simulink model "fxpdemo_probe"  (Simulink 7.6)
settings: Solver=ode45  StartTime=0.0  StopTime=10.0  RelTol=1e-3
Description:
  | Fixed-Point S-Functions: Querying Properties
  | 
  | This model includes more than a dozen examples of S-functions used to probe signal properties.
  | Use this model for simulation only; it does not support code generation.
settings Model: Creator=The MathWorks Inc.  ExtModeAutoUpdateStatusClock=off
settings DataIOCC: SignalLoggingName=logsOut
settings OptimizationCC: InlineInvariantSignals=on  InitFltsAndDblsToZero=on
settings DebuggingCC: SignalResolutionControl=TryResolveAllWithWarning  SolverPrmCheckMsg=none  MultiTaskDSMMsg=warning  MultiTaskCondExecSysMsg=none  SigSpecEnsureSampleTimeMsg=none  StrictBusMsg=None
settings HardwareCC: TargetUnknown=on
settings RTWCC: IncludeERTFirstTime=on

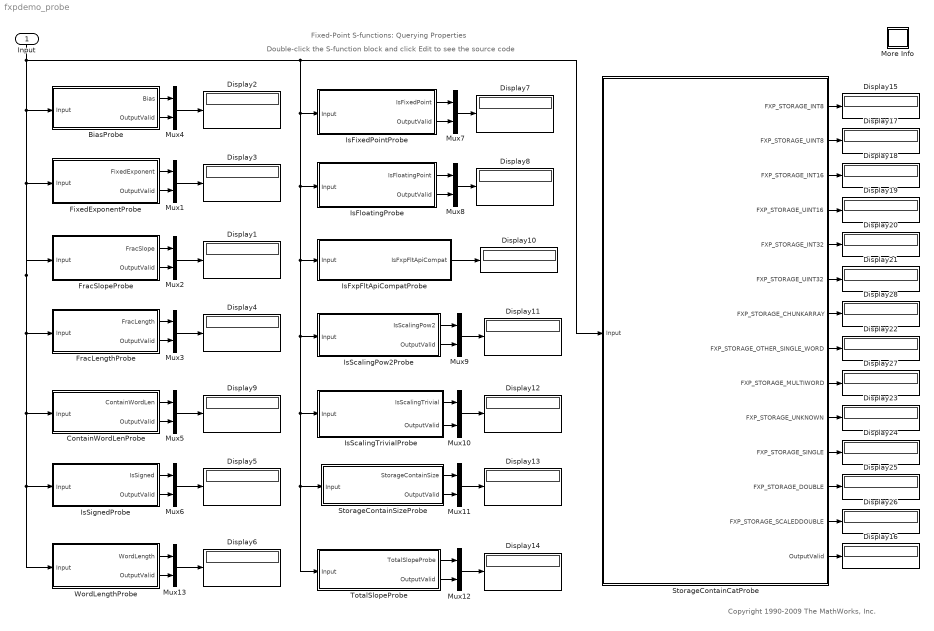
== system fxpdemo_probe ==
  note: Fixed-Point S-functions: Querying Properties
  note: Double-click the S-function block and click Edit to see the source code
  note: Copyright 1990-2009 The MathWorks, Inc.
  Input : Inport  OutDataTypeStr=fixdt(1, 33, 1.1*2^-3,10)
  BiasProbe : Subsystem
  ContainWordLenProbe : Subsystem
  Display{1..28} (28 alike) : Display
  FixedExponentProbe : Subsystem
  FracLengthProbe : Subsystem
  FracSlopeProbe : Subsystem
  IsFixedPointProbe : Subsystem
  IsFloatingProbe : Subsystem
  IsFxpFltApiCompatProbe : Subsystem
  IsScalingPow2Probe : Subsystem
  IsScalingTrivialProbe : Subsystem
  IsSignedProbe : Subsystem
  More Info : Subsystem
      settings: OpenFcn=showdemo(bdroot(gcs))
      mask Display: disp('?')
  Mux{1..13} (13 alike) : Mux  Inputs=2
  StorageContainCatProbe : Subsystem
  StorageContainSizeProbe : Subsystem
  "TotalSlopeProbe " : Subsystem
  WordLengthProbe : Subsystem
  wires:
  Mux5/1 -> Display9/1
  Mux3/1 -> Display4/1
  Mux2/1 -> Display1/1
  Mux1/1 -> Display3/1
  Mux4/1 -> Display2/1
  Input/1 -> FixedExponentProbe/1(Input), BiasProbe/1(Input), IsFixedPointProbe/1(Input), IsFloatingProbe/1(Input), IsFxpFltApiCompatProbe/1(Input), IsScalingPow2Probe/1(Input), IsScalingTrivialProbe/1(Input), StorageContainSizeProbe/1(Input), "TotalSlopeProbe "/1(Input), StorageContainCatProbe/1(Input), FracSlopeProbe/1(Input), FracLengthProbe/1(Input), ContainWordLenProbe/1(Input), IsSignedProbe/1(Input), WordLengthProbe/1(Input)
  Mux6/1 -> Display5/1
  IsSignedProbe/1(IsSigned) -> Mux6/1
  IsSignedProbe/2(OutputValid) -> Mux6/2
  Mux13/1 -> Display6/1
  WordLengthProbe/1(WordLength) -> Mux13/1
  WordLengthProbe/2(OutputValid) -> Mux13/2
  Mux7/1 -> Display7/1
  IsFixedPointProbe/1(IsFixedPoint) -> Mux7/1
  IsFixedPointProbe/2(OutputValid) -> Mux7/2
  IsFloatingProbe/1(IsFloatingPoint) -> Mux8/1
  IsFloatingProbe/2(OutputValid) -> Mux8/2
  IsFxpFltApiCompatProbe/1(IsFxpFltApiCompat) -> Display10/1
  Mux9/1 -> Display11/1
  IsScalingPow2Probe/1(IsScalingPow2) -> Mux9/1
  IsScalingPow2Probe/2(OutputValid) -> Mux9/2
  Mux10/1 -> Display12/1
  IsScalingTrivialProbe/1(IsScalingTrivial) -> Mux10/1
  Mux11/1 -> Display13/1
  StorageContainSizeProbe/1(StorageContainSize) -> Mux11/1
  StorageContainSizeProbe/2(OutputValid) -> Mux11/2
  Mux12/1 -> Display14/1
  "TotalSlopeProbe "/1(TotalSlopeProbe) -> Mux12/1
  "TotalSlopeProbe "/2(OutputValid) -> Mux12/2
  BiasProbe/1(Bias) -> Mux4/1
  BiasProbe/2(OutputValid) -> Mux4/2
  FixedExponentProbe/1(FixedExponent) -> Mux1/1
  FixedExponentProbe/2(OutputValid) -> Mux1/2
  FracSlopeProbe/1(FracSlope) -> Mux2/1
  FracSlopeProbe/2(OutputValid) -> Mux2/2
  FracLengthProbe/1(FracLength) -> Mux3/1
  FracLengthProbe/2(OutputValid) -> Mux3/2
  ContainWordLenProbe/1(ContainWordLen) -> Mux5/1
  ContainWordLenProbe/2(OutputValid) -> Mux5/2
  Mux8/1 -> Display8/1
  IsScalingTrivialProbe/2(OutputValid) -> Mux10/2
  StorageContainCatProbe/1(FXP_STORAGE_INT8) -> Display15/1
  StorageContainCatProbe/2(FXP_STORAGE_UINT8) -> Display17/1
  StorageContainCatProbe/3(FXP_STORAGE_INT16) -> Display18/1
  StorageContainCatProbe/4(FXP_STORAGE_UINT16) -> Display19/1
  StorageContainCatProbe/5(FXP_STORAGE_INT32) -> Display20/1
  StorageContainCatProbe/6(FXP_STORAGE_UINT32) -> Display21/1
  StorageContainCatProbe/8(FXP_STORAGE_OTHER_SINGLE_WORD) -> Display22/1
  StorageContainCatProbe/10(FXP_STORAGE_UNKNOWN) -> Display23/1
  StorageContainCatProbe/11(FXP_STORAGE_SINGLE) -> Display24/1
  StorageContainCatProbe/12(FXP_STORAGE_DOUBLE) -> Display25/1
  StorageContainCatProbe/13(FXP_STORAGE_SCALEDDOUBLE) -> Display26/1
  StorageContainCatProbe/14(OutputValid) -> Display16/1
  StorageContainCatProbe/9(FXP_STORAGE_MULTIWORD) -> Display27/1
  StorageContainCatProbe/7(FXP_STORAGE_CHUNKARRAY) -> Display28/1

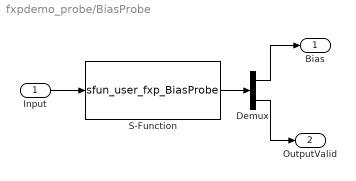
== system fxpdemo_probe/BiasProbe ==
  Input : Inport
  Demux : Demux  Outputs=2
  S-Function : S-Function  FunctionName=sfun_user_fxp_BiasProbe  EnableBusSupport=off
  Bias : Outport
  OutputValid : Outport  Port=2
  wires:
  Input/1 -> S-Function/1
  S-Function/1 -> Demux/1
  Demux/1 -> Bias/1
  Demux/2 -> OutputValid/1

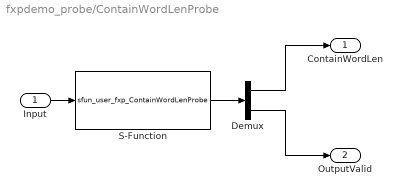
== system fxpdemo_probe/ContainWordLenProbe ==
  Input : Inport
  Demux : Demux  Outputs=2
  S-Function : S-Function  FunctionName=sfun_user_fxp_ContainWordLenProbe  EnableBusSupport=off
  ContainWordLen : Outport
  OutputValid : Outport  Port=2
  wires:
  Demux/1 -> ContainWordLen/1
  Demux/2 -> OutputValid/1
  S-Function/1 -> Demux/1
  Input/1 -> S-Function/1

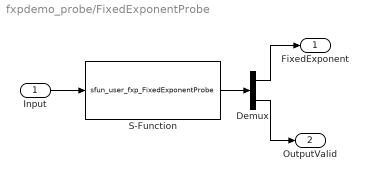
== system fxpdemo_probe/FixedExponentProbe ==
  Input : Inport
  Demux : Demux  Outputs=2
  S-Function : S-Function  FunctionName=sfun_user_fxp_FixedExponentProbe  EnableBusSupport=off
  FixedExponent : Outport
  OutputValid : Outport  Port=2
  wires:
  Demux/2 -> OutputValid/1
  Demux/1 -> FixedExponent/1
  S-Function/1 -> Demux/1
  Input/1 -> S-Function/1

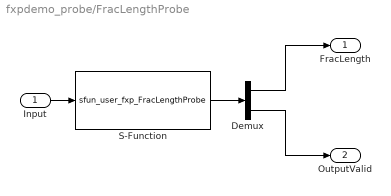
== system fxpdemo_probe/FracLengthProbe ==
  Input : Inport
  Demux : Demux  Outputs=2
  S-Function : S-Function  FunctionName=sfun_user_fxp_FracLengthProbe  EnableBusSupport=off
  FracLength : Outport
  OutputValid : Outport  Port=2
  wires:
  Input/1 -> S-Function/1
  S-Function/1 -> Demux/1
  Demux/2 -> OutputValid/1
  Demux/1 -> FracLength/1

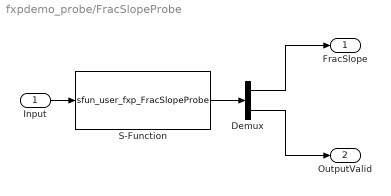
== system fxpdemo_probe/FracSlopeProbe ==
  Input : Inport
  Demux : Demux  Outputs=2
  S-Function : S-Function  FunctionName=sfun_user_fxp_FracSlopeProbe  EnableBusSupport=off
  FracSlope : Outport
  OutputValid : Outport  Port=2
  wires:
  Demux/1 -> FracSlope/1
  Demux/2 -> OutputValid/1
  S-Function/1 -> Demux/1
  Input/1 -> S-Function/1

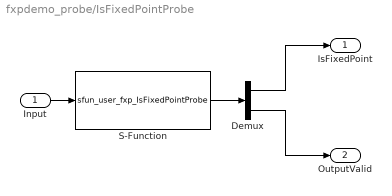
== system fxpdemo_probe/IsFixedPointProbe ==
  Input : Inport
  Demux : Demux  Outputs=2
  S-Function : S-Function  FunctionName=sfun_user_fxp_IsFixedPointProbe  EnableBusSupport=off
  IsFixedPoint : Outport
  OutputValid : Outport  Port=2
  wires:
  Input/1 -> S-Function/1
  S-Function/1 -> Demux/1
  Demux/2 -> OutputValid/1
  Demux/1 -> IsFixedPoint/1

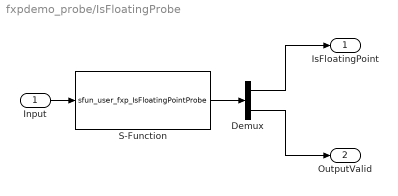
== system fxpdemo_probe/IsFloatingProbe ==
  Input : Inport
  Demux : Demux  Outputs=2
  S-Function : S-Function  FunctionName=sfun_user_fxp_IsFloatingPointProbe  EnableBusSupport=off
  IsFloatingPoint : Outport
  OutputValid : Outport  Port=2
  wires:
  Demux/1 -> IsFloatingPoint/1
  Demux/2 -> OutputValid/1
  S-Function/1 -> Demux/1
  Input/1 -> S-Function/1

== system fxpdemo_probe/IsFxpFltApiCompatProbe ==
  Input : Inport
  S-Function : S-Function  FunctionName=sfun_user_fxp_IsFxpFltApiCompatProbe  EnableBusSupport=off
  IsFxpFltApiCompat : Outport
  wires:
  Input/1 -> S-Function/1
  S-Function/1 -> IsFxpFltApiCompat/1

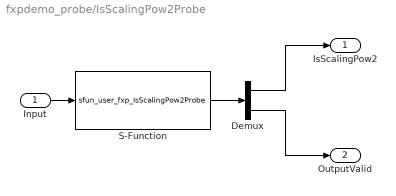
== system fxpdemo_probe/IsScalingPow2Probe ==
  Input : Inport
  Demux : Demux  Outputs=2
  S-Function : S-Function  FunctionName=sfun_user_fxp_IsScalingPow2Probe  EnableBusSupport=off
  IsScalingPow2 : Outport
  OutputValid : Outport  Port=2
  wires:
  Input/1 -> S-Function/1
  S-Function/1 -> Demux/1
  Demux/2 -> OutputValid/1
  Demux/1 -> IsScalingPow2/1

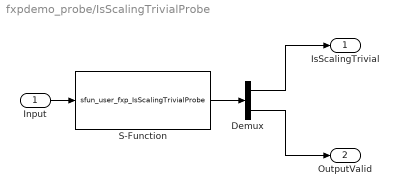
== system fxpdemo_probe/IsScalingTrivialProbe ==
  Input : Inport
  Demux : Demux  Outputs=2
  S-Function : S-Function  FunctionName=sfun_user_fxp_IsScalingTrivialProbe  EnableBusSupport=off
  IsScalingTrivial : Outport
  OutputValid : Outport  Port=2
  wires:
  Demux/1 -> IsScalingTrivial/1
  Demux/2 -> OutputValid/1
  S-Function/1 -> Demux/1
  Input/1 -> S-Function/1

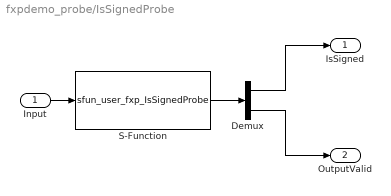
== system fxpdemo_probe/IsSignedProbe ==
  Input : Inport
  Demux : Demux  Outputs=2
  S-Function : S-Function  FunctionName=sfun_user_fxp_IsSignedProbe  EnableBusSupport=off
  IsSigned : Outport
  OutputValid : Outport  Port=2
  wires:
  Input/1 -> S-Function/1
  S-Function/1 -> Demux/1
  Demux/2 -> OutputValid/1
  Demux/1 -> IsSigned/1

== system fxpdemo_probe/More Info ==

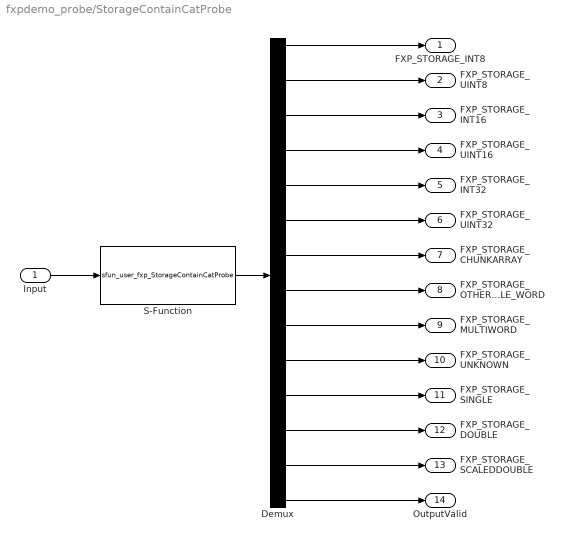
== system fxpdemo_probe/StorageContainCatProbe ==
  Input : Inport
  Demux : Demux  Outputs=14
  S-Function : S-Function  FunctionName=sfun_user_fxp_StorageContainCatProbe  EnableBusSupport=off
  FXP_STORAGE_INT8 : Outport
  FXP_STORAGE_UINT8 : Outport  Port=2
  FXP_STORAGE_INT16 : Outport  Port=3
  FXP_STORAGE_UINT16 : Outport  Port=4
  FXP_STORAGE_INT32 : Outport  Port=5
  FXP_STORAGE_UINT32 : Outport  Port=6
  FXP_STORAGE_CHUNKARRAY : Outport  Port=7
  FXP_STORAGE_OTHER_SINGLE_WORD : Outport  Port=8
  FXP_STORAGE_MULTIWORD : Outport  Port=9
  FXP_STORAGE_UNKNOWN : Outport  Port=10
  FXP_STORAGE_SINGLE : Outport  Port=11
  FXP_STORAGE_DOUBLE : Outport  Port=12
  FXP_STORAGE_SCALEDDOUBLE : Outport  Port=13
  OutputValid : Outport  Port=14
  wires:
  Input/1 -> S-Function/1
  S-Function/1 -> Demux/1
  Demux/2 -> FXP_STORAGE_UINT8/1
  Demux/1 -> FXP_STORAGE_INT8/1
  Demux/3 -> FXP_STORAGE_INT16/1
  Demux/4 -> FXP_STORAGE_UINT16/1
  Demux/5 -> FXP_STORAGE_INT32/1
  Demux/6 -> FXP_STORAGE_UINT32/1
  Demux/7 -> FXP_STORAGE_CHUNKARRAY/1
  Demux/8 -> FXP_STORAGE_OTHER_SINGLE_WORD/1
  Demux/9 -> FXP_STORAGE_MULTIWORD/1
  Demux/10 -> FXP_STORAGE_UNKNOWN/1
  Demux/11 -> FXP_STORAGE_SINGLE/1
  Demux/12 -> FXP_STORAGE_DOUBLE/1
  Demux/13 -> FXP_STORAGE_SCALEDDOUBLE/1
  Demux/14 -> OutputValid/1

== system fxpdemo_probe/StorageContainSizeProbe ==
  Input : Inport
  Demux : Demux  Outputs=2
  S-Function : S-Function  FunctionName=sfun_user_fxp_StorageContainSizeProbe  EnableBusSupport=off
  StorageContainSize : Outport
  OutputValid : Outport  Port=2
  wires:
  Input/1 -> S-Function/1
  S-Function/1 -> Demux/1
  Demux/2 -> OutputValid/1
  Demux/1 -> StorageContainSize/1

== system fxpdemo_probe/TotalSlopeProbe  ==
  Input : Inport
  Demux : Demux  Outputs=2
  S-Function : S-Function  FunctionName=sfun_user_fxp_TotalSlopeProbe  EnableBusSupport=off
  TotalSlopeProbe : Outport
  OutputValid : Outport  Port=2
  wires:
  Demux/1 -> TotalSlopeProbe/1
  Demux/2 -> OutputValid/1
  S-Function/1 -> Demux/1
  Input/1 -> S-Function/1

== system fxpdemo_probe/WordLengthProbe ==
  Input : Inport
  Demux : Demux  Outputs=2
  S-Function : S-Function  FunctionName=sfun_user_fxp_WordLengthProbe  EnableBusSupport=off
  WordLength : Outport
  OutputValid : Outport  Port=2
  wires:
  Demux/1 -> WordLength/1
  Demux/2 -> OutputValid/1
  S-Function/1 -> Demux/1
  Input/1 -> S-Function/1
